simulink subsystem "RegulatorRobustCont_SubSystem"  (R2020b)
settings: Solver=VariableStepAuto  StartTime=0.0  StopTime=10.0  RelTol=1e-3
values from neighbouring files (symbols this model uses):
  A0 = A22 - L*A12    [StateSpaceControllerNominalCont.m]    (also in StateSpaceControllerNominalDigital.m; StateSpaceControllerRobustCont.m; StateSpaceControllerRobustDigital.m)
  B0 = [B2 - L*B1,(A22 - L*A12)*L+A21-L*A11]    [StateSpaceControllerNominalCont.m]    (also in StateSpaceControllerNominalDigital.m; StateSpaceControllerRobustCont.m; StateSpaceControllerRobustDigital.m)
  C = [1,0]    [StateSpaceControllerNominalCont.m]    (also in StateSpaceControllerNominalDigital.m; StateSpaceControllerNominalDirectDigital.m; StateSpaceControllerRobustCont.m; StateSpaceControllerRobustDigital.m)
  C0 = T*[zeros(pOutput,size(A,1) - pOutput);eye(size(A,1) - pOutput)]    [StateSpaceControllerNominalCont.m]    (also in StateSpaceControllerNominalDigital.m; StateSpaceControllerRobustCont.m; StateSpaceControllerRobustDigital.m)
  D0 = T*[zeros(pOutput,mInput),eye(pOutput);         zeros(size(A,1) - pOutput,mInput),L]    [StateSpaceControllerNominalCont.m]    (also in StateSpaceControllerNominalDigital.m; StateSpaceControllerRobustCont.m; StateSpaceControllerRobustDigital.m)
  Ke = Ke_4    [StateSpaceControllerRobustCont.m]    (also in StateSpaceControllerRobustDigital.m; StateSpaceControllerRobustDirectDigital.m = place(Phie,Gammae,p))
  Nu = reshape(Nu,[],1)    [StateSpaceControllerNominalCont.m]    (also in StateSpaceControllerNominalDigital.m; StateSpaceControllerNominalDirectDigital.m; StateSpaceControllerRobustCont.m; StateSpaceControllerRobustDigital.m)
  Nx = reshape(Nx,[],1)    [StateSpaceControllerNominalCont.m]    (also in StateSpaceControllerNominalDigital.m; StateSpaceControllerNominalDirectDigital.m; StateSpaceControllerRobustCont.m; StateSpaceControllerRobustDigital.m)
settings Model: Creator=umberto  LastModifiedBy=umbe

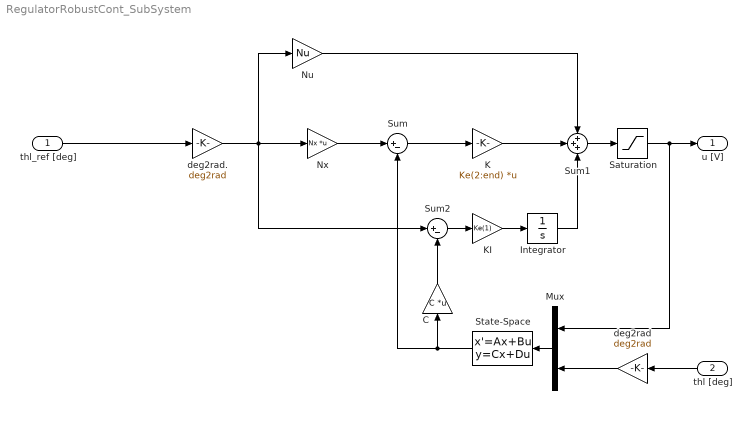
== system RegulatorRobustCont_SubSystem ==
  thl_ref [deg] : Inport
  thl [deg] : Inport  Port=2
  C : Gain  Gain=C  Multiplication=Matrix(K*u)
  Integrator : Integrator
  K : Gain  Gain=Ke(2:end)  Multiplication=Matrix(K*u)
  KI : Gain  Gain=Ke(1)
  Mux : Mux  Inputs=2
  Nu : Gain  Gain=Nu
  Nx : Gain  Gain=Nx  Multiplication=Matrix(K*u)
  Saturation : Saturate  UpperLimit=10  LowerLimit=-10
  State-Space : StateSpace  A=A0  B=B0  C=C0  D=D0  InitialCondition=0
  Sum : Sum  Inputs=|+-
  Sum1 : Sum  Inputs=+++
  Sum2 : Sum  Inputs=|+-
  deg2rad : Gain  Gain=deg2rad
  deg2rad. : Gain  Gain=deg2rad
  u [V] : Outport
  wires:
  deg2rad/1 -> Mux/2
  thl [deg]/1 -> deg2rad/1
  thl_ref [deg]/1 -> deg2rad./1
  deg2rad./1 -> Sum2/1, Nu/1, Nx/1
  Nx/1 -> Sum/1
  Sum/1 -> K/1
  K/1 -> Sum1/2
  Nu/1 -> Sum1/1
  Sum1/1 -> Saturation/1
  Saturation/1 -> u [V]/1, Mux/1
  C/1 -> Sum2/2
  Sum2/1 -> KI/1
  KI/1 -> Integrator/1
  Integrator/1 -> Sum1/3
  Mux/1 -> State-Space/1
  State-Space/1 -> C/1, Sum/2
